simulink model "showcase"  (R2024b)
settings: Solver=FixedStepAuto  StartTime=0.0  StopTime=5  FixedStep=10e-6  RelTol=1e-3
undefined symbols (not defined in the file): DC, p
libraries: DB42S03 x1, mcbpmsmvflib x1
settings Model: Creator=folke  LastModifiedBy=folke

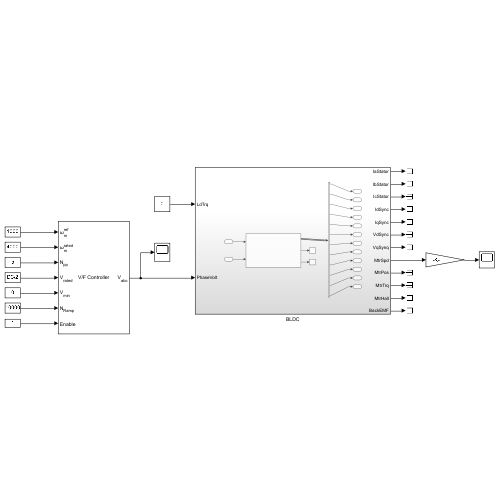
[thumbnail: Simulink's stored preview of the top-level diagram]
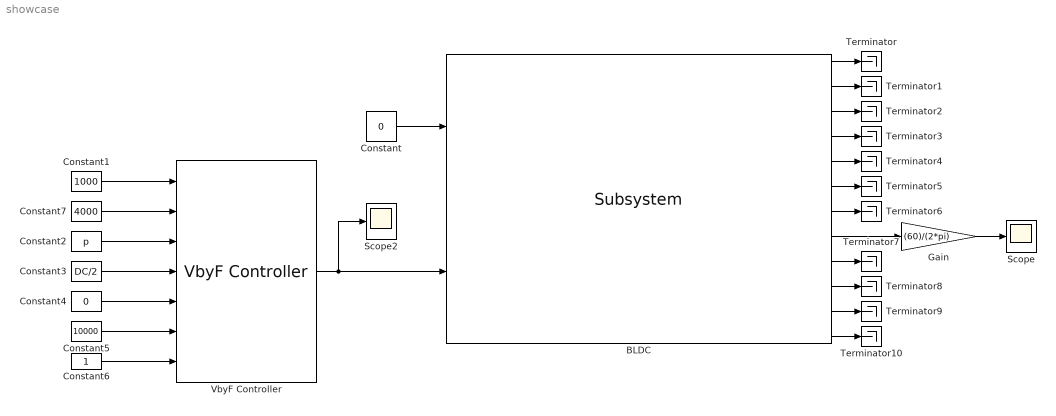
== system showcase ==
  BLDC : DB42S03/Subsystem  SystemSampleTime=-1  VariantActivationTime=update diagram  AllowFlexibleInterface=on  Latency=0  AutoFrameSizeCalculation=off
  Constant : Constant  Value=0
  Constant1 : Constant  Value=1000
  Constant2 : Constant  Value=p
  Constant3 : Constant  Value=DC/2
  Constant4 : Constant  Value=0
  Constant5 : Constant  Value=10000
  Constant6 : Constant
  Constant7 : Constant  Value=4000
  Gain : Gain  Gain=(60)/(2*pi)
  Scope : Scope
  Scope2 : Scope
  Terminator{,1..10} (11 alike) : Terminator
  VbyF Controller : mcbpmsmvflib/VbyF Controller  SpeedUnit=RPM  BaseSpeed=1200  Ts=-1
      settings: LibrarySourceBlock=mcblib/Controls/Controllers/VbyF Controller
  wires:
  Constant/1 -> BLDC/1
  Gain/1 -> Scope/1
  BLDC/8 -> Gain/1
  BLDC/1 -> Terminator/1
  BLDC/2 -> Terminator1/1
  BLDC/3 -> Terminator2/1
  BLDC/4 -> Terminator3/1
  BLDC/5 -> Terminator4/1
  BLDC/6 -> Terminator5/1
  BLDC/7 -> Terminator6/1
  BLDC/9 -> Terminator7/1
  BLDC/10 -> Terminator8/1
  BLDC/11 -> Terminator9/1
  BLDC/12 -> Terminator10/1
  Constant2/1 -> VbyF Controller/3
  Constant3/1 -> VbyF Controller/4
  Constant4/1 -> VbyF Controller/5
  Constant5/1 -> VbyF Controller/6
  Constant6/1 -> VbyF Controller/7
  VbyF Controller/1 -> BLDC/2, Scope2/1
  Constant7/1 -> VbyF Controller/2
  Constant1/1 -> VbyF Controller/1
